simulink model "Lab_4"  (R2021b)
settings: Solver=VariableStepAuto  StartTime=0.0  StopTime=10000  RelTol=1e-3
settings Model: Creator=Саня  LastModifiedBy=Саня

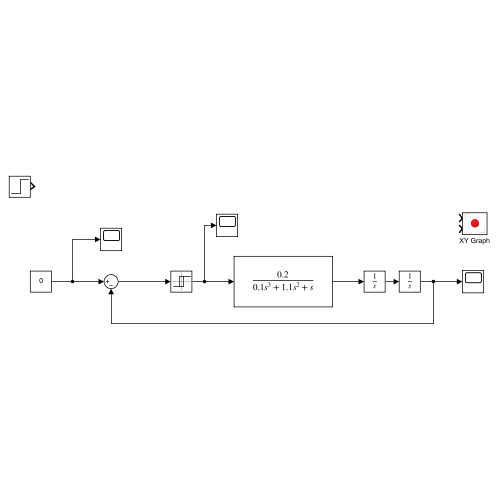
[thumbnail: Simulink's stored preview of the top-level diagram]
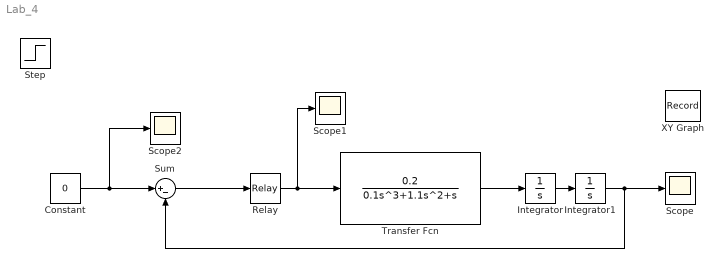
== system Lab_4 ==
  Constant : Constant  Value=0
  Integrator : Integrator  InitialCondition=10
  Integrator1 : Integrator
  Relay : Relay  OnSwitchValue=0  OffSwitchValue=0  OffOutputValue=-1
  Scope : Scope
  Scope1 : Scope
  Scope2 : Scope
  Step : Step  Time=2  After=20  SampleTime=0
  Sum : Sum  Inputs=|+-
  Transfer Fcn : TransferFcn  Numerator=[0.2]  Denominator=[0.1 1.1 1 0]
  XY Graph : Record  FileSettingsInternal="{\"entries\":[{\"content\":{\"excelSettings\":{\"content\":{},\"type\":\"Streamout.ExcelSettings\"}},\"type\":\"Streamout.FileSettingStorage\",\"uuid\":\"e728c376-9073-4c56-997e-e1f49dbd626b\"}],\"packageUris\":[\"http://schema.mathworks.com/mf0/streamout_blocks/R2020a\"],\"version\":\"1.0\"}"  Layout=[1 1]  SignalsInternal="{\"entries\":[{\"content\":{\"signals\":[{\"content\":{\"blockPath\":[\"Lab_4/XY Graph\"],\"channel\":[],\"dimensions\":[1],\"domain\":\"Lab_4/XY Graph\",\"lineColor\":\"#a2142f\",\"plots\":[1],\"port\":1,\"sid\":[],\"signalID\":9},\"type\":\"RecordBlkView.Signal\",\"uuid\":\"5314069b-50dc-43a1-b199-8b87fc39709b\"},{\"content\":{\"blockPath\":[\"Lab_4/XY Graph\"],\"channel\":[],\"dimensions\":[1],\"domain\":\"Lab_4/XY Graph\",\"lineColor\":\"#139fff\",\"plots\":[1],\"port\":2,\"sid\":[],\"signalID\":12},\"type\":\"RecordBlkView.Signal\",\"uuid\":\"2c447a4b-e0a5-45eb-a14e-1b411e345ca5\"}]},\"type\":\"RecordBlkView.InputSignals\",\"uuid\":\"7bf452c2-6645-4108-b5f0-7f3762f2cd38\"}],\"packageUris\":[\"http://schema.mathworks.com/mf0/streamout_blocks/R2020a\"],\"version\":\"1.0\"}"  VisualizationBindings="{\"xyplotplugin\":{\"info\":[{\"series\":[{\"bindingParametersList\":[{\"parameter\":\"X-Axis\",\"signalID\":9,\"signalName\":\"XY Graph:1\"},{\"parameter\":\"Y-Axis\",\"signalID\":12,\"signalName\":\"XY Graph:2\"}],\"seriesID\":30550}],\"subplotID\":1}]}}"  CompatibilityTag=XY
  wires:
  Relay/1 -> Scope1/1, Transfer Fcn/1
  Sum/1 -> Relay/1
  Constant/1 -> Scope2/1, Sum/1
  Transfer Fcn/1 -> Integrator/1
  Integrator/1 -> Integrator1/1
  Integrator1/1 -> Scope/1, Sum/2
